simulink model "descramble"  (R2024b)
settings: Solver=FixedStepAuto  StartTime=0.0  StopTime=10.0  RelTol=1e-3
undefined symbols (not defined in the file): Radix
libraries: dspxfrm3 x2, androidcommunicationlib x2, androidaudiovideolib x1, androiduilib x1, dspsigops x1
settings Model: Creator=hrida  LastModifiedBy=hrida
settings OptimizationCC: DefaultParameterBehavior=Inlined  EnhancedBackFolding=on  PassReuseOutputArgsAs=Individual arguments  ZeroExternalMemoryAtStartup=off  ZeroInternalMemoryAtStartup=off  MaxStackSize=64  OptimizeBlockOrder=speed  DifferentSizesBufferReuse=on  OptimizationCustomize=off  EfficientTunableParamExpr=on
settings DebuggingCC: ParameterTunabilityLossMsg=error
settings HardwareCC: ProdBitPerLong=64  ProdLargestAtomicInteger=LongLong  ProdLargestAtomicFloat=Double  ProdLongLongMode=on  ProdHWDeviceType=ARM Compatible->ARM Cortex-A (64-bit)
settings RTWCC: Description=Embedded Coder  SystemTargetFile=ert.tlc  HardwareBoard=Android Device (64bit)  TLCOptions="-aInlineSetEventsForThisBaseRateFcn=TLC_FALSE -aSuppressMultiTaskScheduler=TLC_FALSE  -aRateBasedStepFcn=0"  TemplateMakefile=ert_default_tmf  RTWVerbose=off  Toolchain=Android SDK/NDK Tools
settings CodeAppCC: ForceParamTrailComments=on  IgnoreCustomStorageClasses=off  OperatorAnnotations=on  SimulinkDataObjDesc=on  SFDataObjDesc=on  InsertBlockDesc=on
settings ERTTargetCC: SupportVariableSizeSignals=on

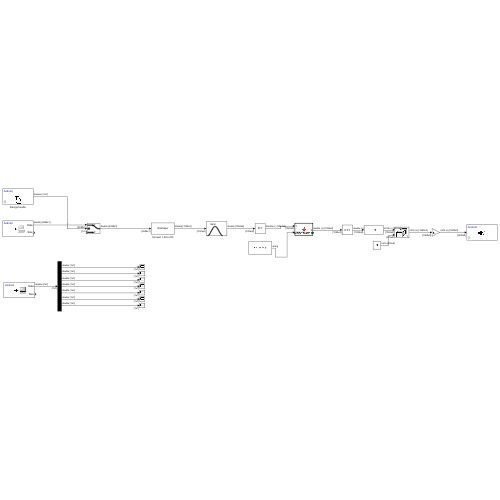
[thumbnail: Simulink's stored preview of the top-level diagram]
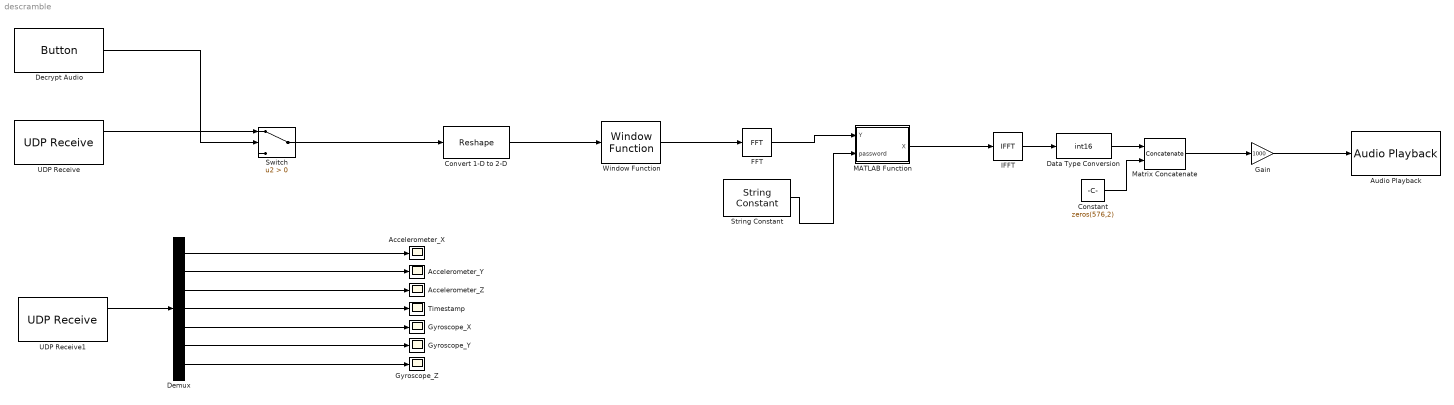
== system descramble ==
  Accelerometer_X : Scope
  Accelerometer_Y : Scope
  Accelerometer_Z : Scope
  Audio Playback : androidaudiovideolib/Audio Playback  SampleFreq=44100  AudioSamplingFreq=44100  SampleTime=0.1  DeviceStr=0  QueueDuration=0  BlockPlatform=Android
  Constant : Constant  Value=zeros(576,2)  VectorParams1D=off  OutDataTypeStr=int16
  Convert 1-D to 2-D : Reshape  OutputDimensionality=Customize  OutputDimensions=[1024 2]
  Data Type Conversion : DataTypeConversion  OutDataTypeStr=int16  SaturateOnIntegerOverflow=off  RndMeth=Floor
  Decrypt Audio : androiduilib/Button  ButtonState=Not pressed  ButtonId=descramble/Decrypt_Audio  State=off  SampleTime=0.1  BlockPlatform=Android
  Demux : Demux  Outputs=7
  FFT : dspxfrm3/FFT  FFTImplementation=Radix-2  CompMethod=Table lookup  TableOpt=NEW  TableOptActive=Speed  BitRevOrder=off  Normalize=off  InheritFFTLength=on  FFTLength=64  WrapInput=on  roundingMode=Ceiling  overflowMode=off  firstCoeffDataTypeStr=Inherit: Same word length as input  firstCoeffLastDataTypeStr=Inherit: Same word length as input  outputMin=[]  outputMax=[]
  Gain : Gain  Gain=1000  ParamDataTypeStr=int16  OutDataTypeStr=int16
  Gyroscope_X : Scope
  Gyroscope_Y : Scope
  Gyroscope_Z : Scope
  IFFT : dspxfrm3/IFFT  FFTImplementation=Radix-2  CompMethod=Table lookup  TableOpt=NEW  TableOptActive=Speed  BitRevOrder=off  cs_in=off  Normalize=on  InheritFFTLength=on  FFTLength=64  WrapInput=on  mode=Real  outSamplingMode=Sample based  roundingMode=Ceiling  overflowMode=off  firstCoeffDataTypeStr=Inherit: Same word length as input  firstCoeffLastDataTypeStr=Inherit: Same word length as input  accumDataTypeStr=Inherit: Same as product output  accumLastDataTypeStr=Inherit: Same as product output  outputMin=[]  outputMax=[]
  MATLAB Function : MATLAB Function  TreatAsAtomicUnit=on
  Matrix Concatenate : Concatenate  Mode=Multidimensional array
  String Constant : StringConstant  String="\"Frequency\""
  Switch : Switch  Criteria=u2 > Threshold  SaturateOnIntegerOverflow=off  InputSameDT=off
  Timestamp : Scope
  UDP Receive : androidcommunicationlib/UDP Receive  localURL='0.0.0.0'  localPort=25000  remoteURL='0.0.0.0'  remotePort=-1  recvBufferSize=8192  signalDatatype=double  dims=2048  isVarSize=off  showBlockingTime=off  blockingTime=0  sampletime=0.1  blockPlatform=Android
  UDP Receive1 : androidcommunicationlib/UDP Receive  localURL='0.0.0.0'  localPort=25001  remoteURL='0.0.0.0'  remotePort=-1  recvBufferSize=8192  signalDatatype=double  dims=7  isVarSize=off  showBlockingTime=off  blockingTime=0  sampletime=0.1  blockPlatform=Android
  Window Function : dspsigops/Window Function  winmode=Apply window to input  wintype=Hann  sampmode=Continuous  samptime=1  N=64  Rs=50  beta=10  winsamp=Symmetric  UserWindow=hamming  OptParams=off  UserParams={'symmetric'}  dataType=double  isSigned=on  wordLen=16  udDataType=sfix(16)  fracBitsMode=Best precision  numFracBits=15  roundingMode=Floor  overflowMode=off  numSidelobes=4  sidelobeLevel=-30
  wires:
  Window Function/1 -> FFT/1
  FFT/1 -> MATLAB Function/1(Y)
  String Constant/1 -> MATLAB Function/2(password)
  MATLAB Function/1(X) -> IFFT/1
  UDP Receive1/1 -> Demux/1
  Demux/1 -> Accelerometer_X/1
  Demux/2 -> Accelerometer_Y/1
  Demux/3 -> Accelerometer_Z/1
  Demux/4 -> Timestamp/1
  Demux/5 -> Gyroscope_X/1
  Demux/6 -> Gyroscope_Y/1
  Demux/7 -> Gyroscope_Z/1
  Decrypt Audio/1 -> Switch/2
  UDP Receive/1 -> Switch/1
  Convert 1-D to 2-D/1 -> Window Function/1
  Switch/1 -> Convert 1-D to 2-D/1
  IFFT/1 -> Data Type Conversion/1
  Constant/1 -> Matrix Concatenate/2
  Matrix Concatenate/1 -> Gain/1
  Gain/1 -> Audio Playback/1
  Data Type Conversion/1 -> Matrix Concatenate/1

== matlab function descramble/MATLAB Function ==
  data: Y input; X output; password input
function X = frequency_descrambling(Y,password)

    N = length(Y);          % FFT size (should be 1024)
    halfN = N/2;            % 512

    % Key regeneration
    seed = sum(double(char(password))) + length(password);
    rng(seed);
    key = randperm(halfN-1) + 1;   % indices 2..512

    % Inverse permutation (size = halfN)
    inv_key = zeros(1, halfN);
    inv_key(key) = 2:halfN;

    % Allocate output as complex
    X = complex(zeros(size(Y)));

    % Preserve DC & Nyquist
    X(1) = Y(1);
    X(halfN+1) = Y(halfN+1);

    % Apply inverse permutation
    X(2:halfN) = Y(inv_key(2:halfN));

    % Restore symmetry
    X(halfN+2:N) = conj(flipud(X(2:halfN)));

end
